simulink model "sim_pos_dist_obs_tcyb"  (R2020a)
settings: Solver=ode4  StartTime=0.0  StopTime=30.0  FixedStep=0.01  RelTol=1e-3
values from neighbouring files (symbols this model uses):
  alfa_theta = 20    [draw_compare_dist_pos_obs.m]
  alfa_theta_obs = 100    [draw_compare_dist_pos_obs.m]
  beta1 = 1.2    [draw_compare_dist_pos_obs.m]
  beta2 = 0.8    [draw_compare_dist_pos_obs.m]
  delta_p_i_0 = zeros(3, NF)    [draw_compare_dist_pos_obs.m]
  delta_v_i_0 = zeros(3, NF)    [draw_compare_dist_pos_obs.m]
  dp_aa_t = 0.2 * ones(3, 5) + ( 1.0 - 0.2 ) * rand(3, 5)    [draw_compare_dist_pos_obs.m]
  dp_ff_t = [ 0.4 * ones(1, 5) + ( 1.0 - 0.4 ) * rand(1, 5);                      0.4 * ones(1, 5) + ( 1.0 - 0.4 ) * rand(1, 5);                      0.2 * ones(1, 5) + ( 0.6 - 0.2 ) * rand(1, 5) ]    [draw_compare_dist_pos_obs.m]
  dp_phi_t = ( - pi / 2 ) * ones(3, 5) + ( pi / 2 - ( - pi / 2 ) ) * rand(3, 5)    [draw_compare_dist_pos_obs.m]
  eps_zeta = 0.2    [draw_compare_dist_pos_obs.m]
  etai_0 = zeros(3,5)    [draw_compare_dist_pos_obs.m]
  gamma_obs_1 = 4    [draw_compare_dist_pos_obs.m]
  gamma_obs_2 = 4    [draw_compare_dist_pos_obs.m]
  kai_1_t = 0.02    [draw_compare_dist_pos_obs.m]
  kai_3_t = 0.1    [draw_compare_dist_pos_obs.m]
  kai_chi_1 = diag([6; 6; 6])    [draw_compare_dist_pos_obs.m]
  kai_chi_2 = diag([6; 6; 6])    [draw_compare_dist_pos_obs.m]
  kai_u_1 = diag([8; 8; 8])    [draw_compare_dist_pos_obs.m]
  kai_u_2 = diag([8; 8; 8])    [draw_compare_dist_pos_obs.m]
  ksii_0 = zeros(3,5)    [draw_compare_dist_pos_obs.m]
  l1v = diag([20; 20; 20])    [draw_compare_dist_pos_obs.m]
  l2v = diag([30; 30; 30])    [draw_compare_dist_pos_obs.m]
  mass_i = zeros(1,NF)    [draw_compare_dist_pos_obs.m]
  Mii = diag([1;0;0;0;1])    [draw_compare_dist_pos_obs.m]
  pos0 = zeros(3, 1)    [draw_compare_dist_pos_obs.m]
  PZ0 = P0(3)    [draw_compare_dist_pos_obs.m]
  PZ1 = 10    [draw_compare_dist_pos_obs.m]
  Qci_init = repmat([1;0;0;0],1,NF)    [draw_compare_dist_pos_obs.m]
  R0 = 4    [draw_compare_dist_pos_obs.m]
  R1 = 8    [draw_compare_dist_pos_obs.m]
  Rx2 = 10    [draw_compare_dist_pos_obs.m]
  Ry2 = 6    [draw_compare_dist_pos_obs.m]
  Rz2 = 4    [draw_compare_dist_pos_obs.m]
  T0 = 0    [draw_compare_dist_pos_obs.m]
  T1 = tseq1    (= 10)    [draw_compare_dist_pos_obs.m]
  T12 = tseq1 + tseq12    (= 20)    [draw_compare_dist_pos_obs.m]
  T2 = tseq1 + tseq12 + tseq2    (= 30)    [draw_compare_dist_pos_obs.m]
  tf2_zeta = 2    [draw_compare_dist_pos_obs.m]
  theta0 = ( 2 / 5 ) * pi    (= 1.25663706144)    [draw_compare_dist_pos_obs.m]
  vel0 = zeros(3, 1)    [draw_compare_dist_pos_obs.m]
  Wij = [0,0,1,0,0;              0,0,1,1,0;              1,0,0,0,1;              0,1,1,0,0;              0,0,1,0,0]    [draw_compare_dist_pos_obs.m]
  X1 = 8    [draw_compare_dist_pos_obs.m]
  X2 = 2    [draw_compare_dist_pos_obs.m]
  X3 = 3    [draw_compare_dist_pos_obs.m]
  Y1 = 10    [draw_compare_dist_pos_obs.m]
  Y2 = 2    [draw_compare_dist_pos_obs.m]
  Y3 = 4    [draw_compare_dist_pos_obs.m]
  Z1 = 4    [draw_compare_dist_pos_obs.m]
  Z2 = -6    [draw_compare_dist_pos_obs.m]
  Z3 = 2    [draw_compare_dist_pos_obs.m]
undefined symbols (not defined in the file or in its folder): cal_frac_squ, p_beta1, p_beta2, p_dbeta1, p_dbeta2, p_gamma1_pos, p_gamma1_vel, p_gamma2_pos, p_gamma2_vel, q_beta1, q_beta2, q_dbeta1, q_dbeta2, q_gamma1_pos, q_gamma1_vel, q_gamma2_pos, q_gamma2_vel
(part 4 of 4)

== matlab function sim_pos_dist_obs_tcyb/cal d_theta_err_ksi agent 4 ==
  data: alfa_theta input; beta1 input; d_theta_err_ksi_1_4 output; beta2 input; d_err_ksi_squ_1_node_4 input; d_err_ksi_squ_2_node_4 input; err_ksi_squ_1_node_4 input; err_ksi_squ_2_node_4 input; err_ksi_vec input; d_theta_err_ksi_2_4 output; err_eta_vec input
function [d_theta_err_ksi_1_4, d_theta_err_ksi_2_4] = fcn(alfa_theta, beta1, beta2, d_err_ksi_squ_1_node_4, d_err_ksi_squ_2_node_4, ...
                                                                                                        err_ksi_squ_1_node_4, err_ksi_squ_2_node_4, err_ksi_vec, err_eta_vec)
%%%% 计算平滑递增函数的导数
iiuav = 4;
kk_alfa = alfa_theta;
d_theta_err_ksi_1_4 = ( beta1 .* d_err_ksi_squ_1_node_4(:) .* sign(err_ksi_vec(:,iiuav)) .* ( -1 + 2 ./ ( 1 + exp( -kk_alfa .* err_ksi_vec(:,iiuav) ) ) ) + ...
                                            err_ksi_squ_1_node_4(:) .* ( 2 .* kk_alfa .* exp( -kk_alfa .* err_ksi_vec(:,iiuav) ) ./ ( ( 1 + exp( -kk_alfa .* err_ksi_vec(:,iiuav) ) ) .^ 2) ) ) ...
                                            .* err_eta_vec(:,iiuav);
d_theta_err_ksi_2_4 = ( beta2 .* d_err_ksi_squ_2_node_4(:) .* sign(err_ksi_vec(:,iiuav)) .* ( -1 + 2 ./ ( 1 + exp( -kk_alfa .* err_ksi_vec(:,iiuav) ) ) ) + ...
                                            err_ksi_squ_2_node_4(:) .* ( 2 .* kk_alfa .* exp( -kk_alfa .* err_ksi_vec(:,iiuav) ) ./ ( ( 1 + exp( -kk_alfa .* err_ksi_vec(:,iiuav) ) ) .^ 2) ) ) ...
                                            .* err_eta_vec(:,iiuav);

== matlab function sim_pos_dist_obs_tcyb/choose ksi_est_err 17 ==
  data: x input; y output
function y = fcn(x)
iiuav = 4;
y = x(:,iiuav);

== matlab function sim_pos_dist_obs_tcyb/choose ksi_est_err 18 ==
  data: x input; y output
function y = fcn(x)
iiuav = 4;
y = x(:,iiuav);

== matlab function sim_pos_dist_obs_tcyb/trans to column16 ==
  data: x input; y output
function y = fcn(x)
y = x(:);

== matlab function sim_pos_dist_obs_tcyb/trans to column17 ==
  data: x input; y output
function y = fcn(x)
y = x(:);

== matlab function sim_pos_dist_obs_tcyb/cal abs 19 ==
  data: x input; y output
function y = fcn(x)
y = abs(x(:));

== matlab function sim_pos_dist_obs_tcyb/cal abs 20 ==
  data: x input; y output
function y = fcn(x)
y = abs(x(:));

== matlab function sim_pos_dist_obs_tcyb/cal d_theta_err_ksi agent 5 ==
  data: alfa_theta input; beta1 input; d_theta_err_ksi_1_5 output; beta2 input; d_err_ksi_squ_1_node_5 input; d_err_ksi_squ_2_node_5 input; err_ksi_squ_1_node_5 input; err_ksi_squ_2_node_5 input; err_ksi_vec input; d_theta_err_ksi_2_5 output; err_eta_vec input
function [d_theta_err_ksi_1_5, d_theta_err_ksi_2_5] = fcn(alfa_theta, beta1, beta2, d_err_ksi_squ_1_node_5, d_err_ksi_squ_2_node_5, ...
                                                                                                        err_ksi_squ_1_node_5, err_ksi_squ_2_node_5, err_ksi_vec, err_eta_vec)
%%%% 计算平滑递增函数的导数
iiuav = 5;
kk_alfa = alfa_theta;
d_theta_err_ksi_1_5 = ( beta1 .* d_err_ksi_squ_1_node_5(:) .* sign(err_ksi_vec(:,iiuav)) .* ( -1 + 2 ./ ( 1 + exp( -kk_alfa .* err_ksi_vec(:,iiuav) ) ) ) + ...
                                            err_ksi_squ_1_node_5(:) .* ( 2 .* kk_alfa .* exp( -kk_alfa .* err_ksi_vec(:,iiuav) ) ./ ( ( 1 + exp( -kk_alfa .* err_ksi_vec(:,iiuav) ) ) .^ 2) ) ) ...
                                            .* err_eta_vec(:,iiuav);
d_theta_err_ksi_2_5 = ( beta2 .* d_err_ksi_squ_2_node_5(:) .* sign(err_ksi_vec(:,iiuav)) .* ( -1 + 2 ./ ( 1 + exp( -kk_alfa .* err_ksi_vec(:,iiuav) ) ) ) + ...
                                            err_ksi_squ_2_node_5(:) .* ( 2 .* kk_alfa .* exp( -kk_alfa .* err_ksi_vec(:,iiuav) ) ./ ( ( 1 + exp( -kk_alfa .* err_ksi_vec(:,iiuav) ) ) .^ 2) ) ) ...
                                            .* err_eta_vec(:,iiuav);
